simulink model "sampleModel347"  (R2021b)
settings: Solver=VariableStepAuto  StartTime=0.0  StopTime=10.0  RelTol=1e-3
undefined symbols (not defined in the file or in its folder): DiscIntNeverNeededParam, Newton, Raphson
libraries: simulink x9, slpidlib x1
settings Model: Creator=user  LastModifiedBy=user

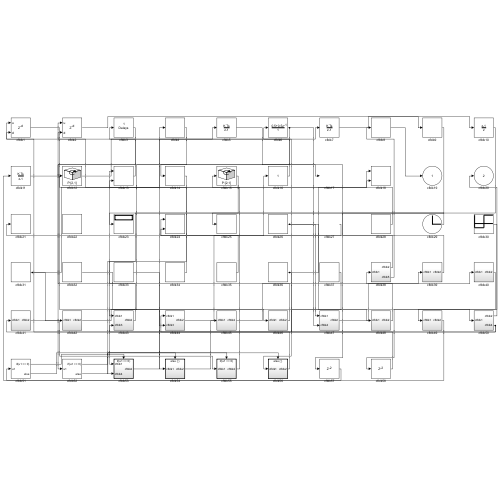
[thumbnail: Simulink's stored preview of the top-level diagram]
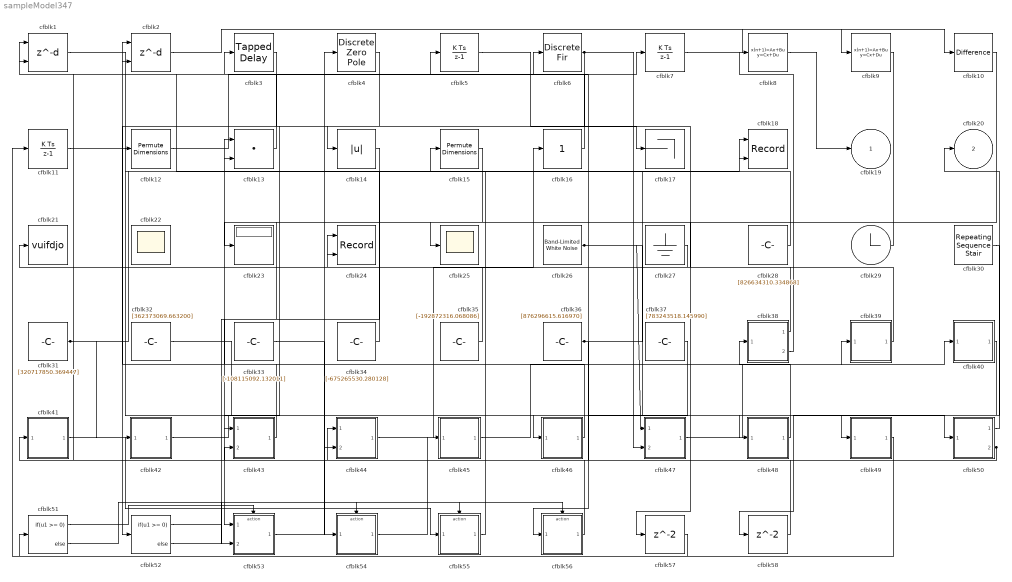
== system sampleModel347 ==
  cfblk1 : Delay  DelayLengthSource=Input port  SampleTime=1
      settings: InputPortMap=u0,p1
  cfblk10 : simulink/Discrete/Difference  ICPrevInput=0.0  OutMin=[]  OutMax=[]  OutDataTypeStr=Inherit: Inherit via back propagation  OutDataType=fixdt(1, 16)  OutScaling=2^-10  DoSatur=off
  cfblk11 : DiscreteIntegrator  ICPrevOutput=DiscIntNeverNeededParam  ICPrevScaledInput=DiscIntNeverNeededParam
  cfblk12 : PermuteDimensions
  cfblk13 : DotProduct  InputSameDT=on  OutDataTypeStr=Inherit: Inherit via internal rule
  cfblk14 : Abs
  cfblk15 : PermuteDimensions
  cfblk16 : simulink/Math Operations/Slider Gain  gain=1  low=0  high=2
  cfblk17 : Terminator
  cfblk18 : Record  FileSettingsInternal="{\"entries\":[{\"content\":{\"excelSettings\":{\"content\":{},\"type\":\"Streamout.ExcelSettings\"}},\"type\":\"Streamout.FileSettingStorage\",\"uuid\":\"55d644a5-12b3-4429-a882-e1257f208ec1\"}],\"packageUris\":[\"http://schema.mathworks.com/mf0/streamout_blocks/R2020a\"],\"version\":\"1.0\"}"  Layout=[1 1]  SignalsInternal="{\"entries\":[{\"content\":{\"signals\":[{\"content\":{\"blockPath\":[\"sampleModel347/cfblk18\"],\"channel\":[],\"dimensions\":[1],\"domain\":\"sampleModel347/cfblk18\",\"lineColor\":\"#a2142f\",\"plots\":[1],\"port\":1,\"sid\":[\"\"],\"signalID\":14541,\"signalName\":\"cfblk36\"},\"type\":\"RecordBlkView.Signal\",\"uuid\":\"b67f685b-2653-4f6a-806c-a94c2618ce46\"},{\"content\":{\"blockPath\":[\"sampleModel347/cfblk18\"],\"channel\":[],\"dimensions\":[1],\"domain\":\"sampleModel347/cfblk18\",\"lineColor\":\"#139fff\",\"plots\":[1],\"port\":2,\"sid\":[\"\"],\"signalID\":14545,\"signalName\":\"cfblk11\"},\"type\":\"RecordBlkView.Signal\",\"uuid\":\"4f3fc5b9-18d0-4829-bc90-462738cc687d\"}]},\"type\":\"RecordBlkView.InputSignals\",\"uuid\":\"f6bcba47-d682-4b72-9895-2afc48cdd87f\"}],\"packageUris\":[\"http://schema.mathworks.com/mf0/streamout_blocks/R2020a\"],\"version\":\"1.0\"}"  VisualizationBindings="{\"xyplotplugin\":{\"info\":[{\"series\":[{\"bindingParametersList\":[{\"parameter\":\"X-Axis\",\"signalID\":14541,\"signalName\":\"cfblk36\"},{\"parameter\":\"Y-Axis\",\"signalID\":14545,\"signalName\":\"cfblk11\"}],\"seriesID\":40911}],\"subplotID\":1}]}}"  CompatibilityTag=XY
  cfblk2 : Delay  DelayLengthSource=Input port  SampleTime=1
      settings: InputPortMap=u0,p1
  cfblk21 : ToWorkspace  VariableName=vuifdjo  SaveFormat=Timeseries  SampleTime=-1
  cfblk22 : Scope
      settings: Floating=on
  cfblk23 : Display
  cfblk24 : Record  FileSettingsInternal="{\"entries\":[{\"content\":{\"excelSettings\":{\"content\":{},\"type\":\"Streamout.ExcelSettings\"}},\"type\":\"Streamout.FileSettingStorage\",\"uuid\":\"c7d4169a-b585-49ac-aca8-b838ce6defab\"}],\"packageUris\":[\"http://schema.mathworks.com/mf0/streamout_blocks/R2020a\"],\"version\":\"1.0\"}"  Layout=[1 1]  SignalsInternal="{\"entries\":[{\"content\":{\"signals\":[{\"content\":{\"blockPath\":[\"sampleModel347/cfblk24\"],\"channel\":[],\"dimensions\":[1],\"domain\":\"sampleModel347/cfblk24\",\"lineColor\":\"#a2142f\",\"plots\":[1],\"port\":1,\"sid\":[\"\"],\"signalID\":14549,\"signalName\":\"cfblk35\"},\"type\":\"RecordBlkView.Signal\",\"uuid\":\"209a5a0c-6ba4-41ae-874b-22178ed96705\"},{\"content\":{\"blockPath\":[\"sampleModel347/cfblk24\"],\"channel\":[],\"dimensions\":[1],\"domain\":\"sampleModel347/cfblk24\",\"lineColor\":\"#139fff\",\"plots\":[1],\"port\":2,\"sid\":[\"\"],\"signalID\":14553,\"signalName\":\"cfblk27\"},\"type\":\"RecordBlkView.Signal\",\"uuid\":\"494a0b99-c67e-416d-8697-a0053402a19d\"}]},\"type\":\"RecordBlkView.InputSignals\",\"uuid\":\"05a8ac8a-22e6-46ac-8d63-08b6bf11da06\"}],\"packageUris\":[\"http://schema.mathworks.com/mf0/streamout_blocks/R2020a\"],\"version\":\"1.0\"}"  VisualizationBindings="{\"xyplotplugin\":{\"info\":[{\"series\":[{\"bindingParametersList\":[{\"parameter\":\"X-Axis\",\"signalID\":14549,\"signalName\":\"cfblk35\"},{\"parameter\":\"Y-Axis\",\"signalID\":14553,\"signalName\":\"cfblk27\"}],\"seriesID\":25638}],\"subplotID\":1}]}}"  CompatibilityTag=XY
  cfblk25 : Scope
  cfblk26 : simulink/Sources/Band-Limited White Noise  Cov=[3794398979.519006]  Ts=0.1  seed=[782136946.000000]
  cfblk27 : Ground
  cfblk28 : Constant  Value=[826634310.334868]  SampleTime=1
  cfblk29 : Clock
  cfblk3 : simulink/Discrete/Tapped Delay  vinit=0.0  samptime=-1  NumDelays=1  DelayOrder=Oldest  includeCurrent=off
  cfblk30 : simulink/Sources/Repeating Sequence Stair  OutValues=[-457308169.608421, 909466912.372640]  tsamp=-1  OutMin=[]  OutMax=[]  OutDataTypeStr=double  OutputDataTypeScalingMode=double  OutDataType=fixdt(0,8)  ConRadixGroup=Best Precision: Vector-wise  OutScaling=2^-12
  cfblk31 : Constant  Value=[320717850.369447]  SampleTime=1
  cfblk32 : Constant  Value=[362373069.663200]  SampleTime=1
  cfblk33 : Constant  Value=[-108115092.132011]  SampleTime=1
  cfblk34 : Constant  Value=[-675265530.280128]  SampleTime=1
  cfblk35 : Constant  Value=[-192872316.068086]  SampleTime=1
  cfblk36 : Constant  Value=[876296615.616970]  SampleTime=1
  cfblk37 : Constant  Value=[783243518.145990]  SampleTime=1
  cfblk38 : Subsystem
  cfblk39 : Subsystem
  cfblk4 : DiscreteZeroPole  Poles=[0 0.5]  Gain=1
  cfblk40 : Subsystem
  cfblk41 : Subsystem
  cfblk42 : Subsystem
  cfblk43 : Subsystem
  cfblk44 : Subsystem
  cfblk45 : Subsystem
  cfblk46 : Subsystem
  cfblk47 : Subsystem
  cfblk48 : Subsystem
  cfblk49 : Subsystem
  cfblk5 : DiscreteIntegrator  ICPrevOutput=DiscIntNeverNeededParam  ICPrevScaledInput=DiscIntNeverNeededParam
  cfblk50 : Subsystem
  cfblk51 : If  IfExpression=u1 >= 0  SampleTime=1
  cfblk52 : If  IfExpression=u1 >= 0  SampleTime=1
  cfblk53 : Subsystem  TreatAsAtomicUnit=on
  cfblk54 : Subsystem  TreatAsAtomicUnit=on
  cfblk55 : Subsystem  TreatAsAtomicUnit=on
  cfblk56 : Subsystem  TreatAsAtomicUnit=on
  cfblk57 : Delay  SampleTime=1
  cfblk58 : Delay  SampleTime=1
  cfblk6 : DiscreteFir  SampleTime=1
  cfblk7 : DiscreteIntegrator  ICPrevOutput=DiscIntNeverNeededParam  ICPrevScaledInput=DiscIntNeverNeededParam
  cfblk8 : DiscreteStateSpace
  cfblk9 : DiscreteStateSpace
  cfblk19 : Outport
  cfblk20 : Outport  Port=2
  wires:
  cfblk32/1 -> cfblk46/1(cfblk1)
  cfblk15/1 -> cfblk25/1
  cfblk37/1 -> cfblk44/1(cfblk1)
  cfblk35/1 -> cfblk24/1
  cfblk27/1 -> cfblk24/2
  cfblk38/1(cfblk2) -> cfblk14/1
  cfblk13/1 -> cfblk1/1
  cfblk1/1 -> cfblk44/2(cfblk3)
  cfblk16/1 -> cfblk3/1
  cfblk55/1(cfblk2) -> cfblk15/1
  cfblk36/1 -> cfblk18/1, cfblk56/1(cfblk1)
  cfblk26/1 -> cfblk47/1(cfblk1), cfblk50/1(cfblk1)
  cfblk33/1 -> cfblk54/1(cfblk1)
  cfblk12/1 -> cfblk5/1
  cfblk7/1 -> cfblk10/1
  cfblk4/1 -> cfblk52/1
  cfblk38/2(cfblk5) -> cfblk21/1
  cfblk5/1 -> cfblk17/1
  cfblk49/1(cfblk2) -> cfblk11/1
  cfblk46/1(cfblk2) -> cfblk13/1
  cfblk30/1 -> cfblk49/1(cfblk1)
  cfblk41/1(cfblk2) -> cfblk55/1(cfblk1)
  cfblk6/1 -> cfblk47/2(cfblk4), cfblk43/1(cfblk1)
  cfblk31/1 -> cfblk4/1, cfblk42/1(cfblk1)
  cfblk53/1(cfblk2) -> cfblk7/1
  cfblk39/1(cfblk2) -> cfblk8/1
  cfblk56/1(cfblk2) -> cfblk1/2
  cfblk44/1(cfblk2) -> cfblk16/1
  cfblk8/1 -> cfblk19/1
  cfblk28/1 -> cfblk13/2
  cfblk54/1(cfblk2) -> cfblk45/1(cfblk1)
  cfblk29/1 -> cfblk23/1
  cfblk11/1 -> cfblk18/2
  cfblk47/1(cfblk2) -> cfblk40/1(cfblk1)
  cfblk2/1 -> cfblk9/1
  cfblk43/1(cfblk2) -> cfblk2/1
  cfblk3/1 -> cfblk12/1
  cfblk9/1 -> cfblk53/1(cfblk1)
  cfblk14/1 -> cfblk53/2(cfblk4)
  cfblk42/1(cfblk2) -> cfblk48/1(cfblk1)
  cfblk34/1 -> cfblk2/2
  cfblk48/1(cfblk2) -> cfblk38/1(cfblk1)
  cfblk45/1(cfblk2) -> cfblk39/1(cfblk1)
  cfblk50/1(cfblk2) -> cfblk20/1
  cfblk50/2(cfblk4) -> cfblk41/1(cfblk1), cfblk43/2(cfblk3)
  cfblk51/1 -> cfblk53/Action
  cfblk51/2 -> cfblk54/Action
  cfblk52/1 -> cfblk55/Action
  cfblk52/2 -> cfblk56/Action
  cfblk10/1 -> cfblk57/1
  cfblk57/1 -> cfblk51/1
  cfblk40/1(cfblk2) -> cfblk58/1
  cfblk58/1 -> cfblk6/1

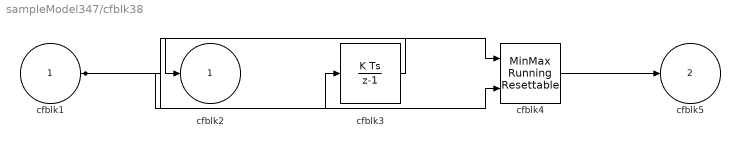
== system sampleModel347/cfblk38 ==
  cfblk1 : Inport
  cfblk3 : DiscreteIntegrator  ICPrevOutput=DiscIntNeverNeededParam  ICPrevScaledInput=DiscIntNeverNeededParam
  cfblk4 : simulink/Math Operations/MinMax Running Resettable  Function=min  vinit=0.0
  cfblk2 : Outport
  cfblk5 : Outport  Port=2
  wires:
  cfblk3/1 -> cfblk2/1
  cfblk1/1 -> cfblk3/1, cfblk4/1, cfblk4/2
  cfblk4/1 -> cfblk5/1

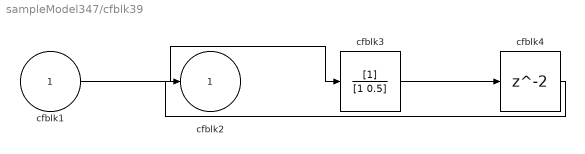
== system sampleModel347/cfblk39 ==
  cfblk1 : Inport
  cfblk3 : DiscreteFilter  SampleTime=1
  cfblk4 : Delay  SampleTime=1
  cfblk2 : Outport
  wires:
  cfblk3/1 -> cfblk4/1
  cfblk1/1 -> cfblk3/1
  cfblk4/1 -> cfblk2/1

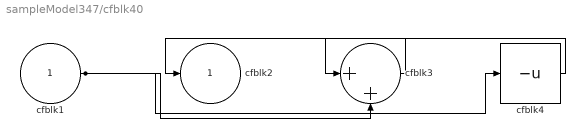
== system sampleModel347/cfblk40 ==
  cfblk1 : Inport
  cfblk3 : Sum  Inputs=|++
  cfblk4 : UnaryMinus
  cfblk2 : Outport
  wires:
  cfblk3/1 -> cfblk2/1
  cfblk1/1 -> cfblk4/1, cfblk3/2
  cfblk4/1 -> cfblk3/1

== system sampleModel347/cfblk41 ==
  cfblk1 : Inport
  cfblk3 : UnaryMinus
  cfblk2 : Outport
  wires:
  cfblk1/1 -> cfblk3/1
  cfblk3/1 -> cfblk2/1

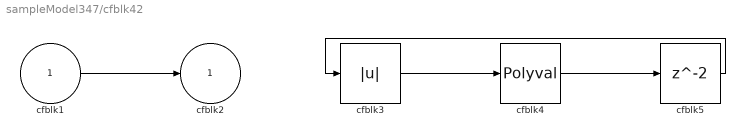
== system sampleModel347/cfblk42 ==
  cfblk1 : Inport
  cfblk3 : Abs
  cfblk4 : Polyval  Coefs=[ +2.081618890e-019, -1.441693666e-014, +4.719686976e-010, -8.536869453e-006, +1.621573104e-001, -8.087801117e+001 ]
  cfblk5 : Delay  SampleTime=1
  cfblk2 : Outport
  wires:
  cfblk1/1 -> cfblk2/1
  cfblk3/1 -> cfblk4/1
  cfblk4/1 -> cfblk5/1
  cfblk5/1 -> cfblk3/1

== system sampleModel347/cfblk43 ==
  cfblk1 : Inport
  cfblk3 : Inport  Port=2
  cfblk2 : Outport
  wires:
  cfblk3/1 -> cfblk2/1

== system sampleModel347/cfblk44 ==
  cfblk1 : Inport
  cfblk3 : Inport  Port=2
  cfblk2 : Outport
  wires:
  cfblk3/1 -> cfblk2/1

== system sampleModel347/cfblk45 ==
  cfblk1 : Inport
  cfblk3 : Sqrt  Operator=rSqrt  AlgorithmType=Newton-Raphson  SaturateOnIntegerOverflow=on
  cfblk2 : Outport
  wires:
  cfblk1/1 -> cfblk3/1
  cfblk3/1 -> cfblk2/1

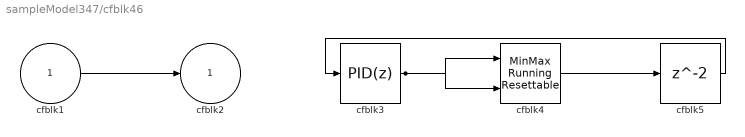
== system sampleModel347/cfblk46 ==
  cfblk1 : Inport
  cfblk3 : slpidlib/PID Controller  Controller=PID  Form=Parallel  TimeDomain=Discrete-time  UseExternalTs=off  SampleTime=1  IntegratorMethod=Forward Euler  FilterMethod=Forward Euler  ControllerParametersSource=internal  P=1  I=1  D=0  UseFilter=on  N=100  TunerSelectOption=Transfer Function Based (PID Tuner App)  InitialConditionSource=internal  InitialConditionForIntegrator=0  InitialConditionForFilter=0  DifferentiatorICPrevScaledInput=0  ExternalReset=none  TrackingMode=off  Kt=1  LimitOutput=off  SatLimitsSource=internal  UpperSaturationLimit=inf  LowerSaturationLimit=-inf  LinearizeAsGain=off  AntiWindupMode=none  Kb=1  POutMin=[]  POutMax=[]  IOutMin=[]  IOutMax=[]  DOutMin=[]  DOutMax=[]  NOutMin=[]  NOutMax=[]  SumOutMin=[]  SumOutMax=[]  SaturationOutMin=[]  SaturationOutMax=[]  PParamMin=[]  PParamMax=[]  IParamMin=[]  IParamMax=[]  DParamMin=[]  DParamMax=[]  NParamMin=[]  NParamMax=[]  KbParamMin=[]  KbParamMax=[]  KtParamMin=[]  KtParamMax=[]  KbOutMin=[]  KbOutMax=[]  KtOutMin=[]  KtOutMax=[]  IntegratorOutMin=[]  IntegratorOutMax=[]  FilterOutMin=[]  FilterOutMax=[]  SumI1OutMin=[]  SumI1OutMax=[]  SumI2OutMin=[]  SumI2OutMax=[]  SumI3OutMin=[]  SumI3OutMax=[]  SumI4OutMin=[]  SumI4OutMax=[]  SumDOutMin=[]  SumDOutMax=[]  DifferentiatorOutMin=[]  DifferentiatorOutMax=[]  FilterDiffOutCoefMin=[]  FilterDiffOutCoefMax=[]  ReciprocalOutMin=[]  ReciprocalOutMax=[]  SumDenOutMin=[]  SumDenOutMax=[]  SumNumOutMin=[]  SumNumOutMax=[]  DivideOutMin=[]  DivideOutMax=[]  UdiffTsProdOutMin=[]  UdiffTsProdOutMax=[]  NTsProdOutMin=[]  NTsProdOutMax=[]  UintegralTsProdOutMin=[]  UintegralTsProdOutMax=[]  UngainTsProdOutMin=[]  UngainTsProdOutMax=[]  IntegratorContinuousStateAttributes=''  IntegratorStateMustResolveToSignalObject=off  IntegratorRTWStateStorageClass=Auto  FilterContinuousStateAttributes=''  FilterStateMustResolveToSignalObject=off  FilterRTWStateStorageClass=Auto  ParallelPVariant=InternalParameters  IdealPVariant=Disabled  IVariant=InternalParameters  DVariant=InternalParameters  IntegratorVariant=Discrete  SatVariant=Disabled  AWVariant=Passthrough  PCopyVariant=Disabled  TRVariant=Disabled  FdbkBlocksVariant=Forward  IdealPFdbkVariant=Disabled  SatFdbkVariant=Disabled  DerivativeFilterVariant=ForwardEulerFilter  NVariant=InternalParameters  NCopyVariant=Disabled  FilterICVariant=InternalICsFilter  IntegratorICVariant=InternalICs  ExternalResetVariant=Disabled  TRSumVariant=Passthrough  SumFdbkVariant=Disabled  SumVariant=Sum_PID  TsampFilterVariant=InternalTs  TsampNgainVariant=Passthrough  TsampIntegralVariant=Passthrough  ExternalSaturationOutDataTypeStr=Inherit: Same as second input
  cfblk4 : simulink/Math Operations/MinMax Running Resettable  Function=min  vinit=0.0
  cfblk5 : Delay  SampleTime=1
  cfblk2 : Outport
  wires:
  cfblk1/1 -> cfblk2/1
  cfblk3/1 -> cfblk4/1, cfblk4/2
  cfblk4/1 -> cfblk5/1
  cfblk5/1 -> cfblk3/1

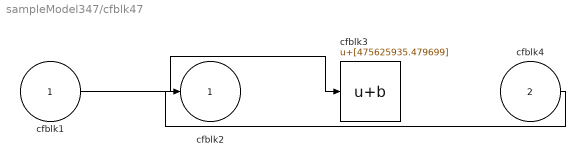
== system sampleModel347/cfblk47 ==
  cfblk1 : Inport
  cfblk4 : Inport  Port=2
  cfblk3 : Bias  Bias=[475625935.479699]
  cfblk2 : Outport
  wires:
  cfblk1/1 -> cfblk3/1
  cfblk4/1 -> cfblk2/1

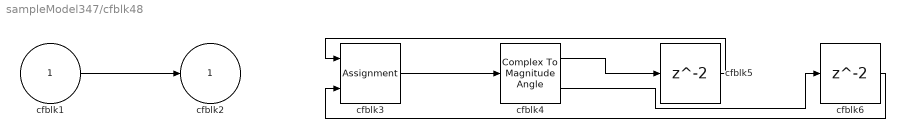
== system sampleModel347/cfblk48 ==
  cfblk1 : Inport
  cfblk3 : Assignment  DiagnosticForDimensions=Warning  IndexOptions=Index vector (dialog)  Indices=1  OutputSizes=1
  cfblk4 : ComplexToMagnitudeAngle
  cfblk5 : Delay  SampleTime=1
  cfblk6 : Delay  SampleTime=1
  cfblk2 : Outport
  wires:
  cfblk1/1 -> cfblk2/1
  cfblk3/1 -> cfblk4/1
  cfblk4/1 -> cfblk5/1
  cfblk5/1 -> cfblk3/1
  cfblk4/2 -> cfblk6/1
  cfblk6/1 -> cfblk3/2

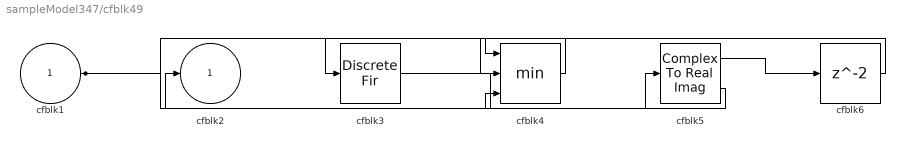
== system sampleModel347/cfblk49 ==
  cfblk1 : Inport
  cfblk3 : DiscreteFir  SampleTime=1
  cfblk4 : MinMax  Inputs=3
  cfblk5 : ComplexToRealImag
  cfblk6 : Delay  SampleTime=1
  cfblk2 : Outport
  wires:
  cfblk5/2 -> cfblk2/1
  cfblk3/1 -> cfblk5/1
  cfblk4/1 -> cfblk3/1
  cfblk1/1 -> cfblk4/2, cfblk4/3
  cfblk5/1 -> cfblk6/1
  cfblk6/1 -> cfblk4/1

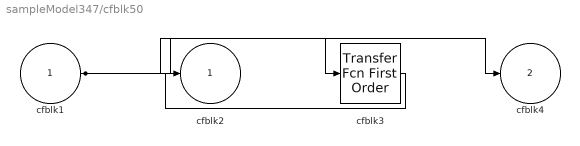
== system sampleModel347/cfblk50 ==
  cfblk1 : Inport
  cfblk3 : simulink/Discrete/Transfer Fcn First Order  PoleZ=0.95  ICPrevOutput=0.0  DoSatur=off
  cfblk2 : Outport
  cfblk4 : Outport  Port=2
  wires:
  cfblk1/1 -> cfblk4/1, cfblk3/1
  cfblk3/1 -> cfblk2/1

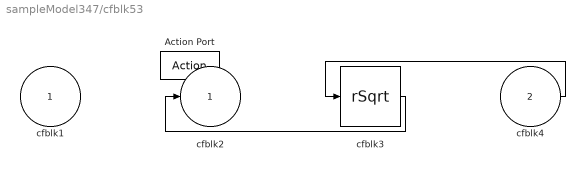
== system sampleModel347/cfblk53 ==
  cfblk1 : Inport
  cfblk4 : Inport  Port=2
  Action Port : ActionPort  ActionPortLabel=if(u1 >= 0)
  cfblk3 : Sqrt  Operator=rSqrt  AlgorithmType=Newton-Raphson  SaturateOnIntegerOverflow=on
  cfblk2 : Outport
  wires:
  cfblk4/1 -> cfblk3/1
  cfblk3/1 -> cfblk2/1

== system sampleModel347/cfblk54 ==
  cfblk1 : Inport
  Action Port : ActionPort  ActionPortLabel=else
  cfblk3 : simulink/Discrete/Tapped Delay  vinit=0.0  samptime=-1  NumDelays=1  DelayOrder=Oldest  includeCurrent=off
  cfblk2 : Outport
  wires:
  cfblk3/1 -> cfblk2/1
  cfblk1/1 -> cfblk3/1

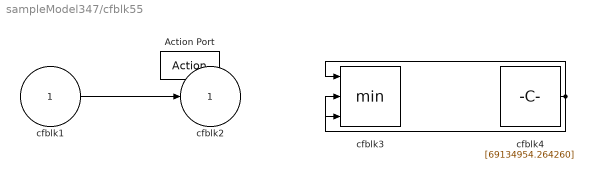
== system sampleModel347/cfblk55 ==
  cfblk1 : Inport
  Action Port : ActionPort  ActionPortLabel=if(u1 >= 0)
  cfblk3 : MinMax  Inputs=3
  cfblk4 : Constant  Value=[69134954.264260]  SampleTime=1
  cfblk2 : Outport
  wires:
  cfblk1/1 -> cfblk2/1
  cfblk4/1 -> cfblk3/1, cfblk3/2, cfblk3/3

== system sampleModel347/cfblk56 ==
  cfblk1 : Inport
  Action Port : ActionPort  ActionPortLabel=else
  cfblk3 : UnitDelay  SampleTime=-1  HasFrameUpgradeWarning=on
  cfblk2 : Outport
  wires:
  cfblk1/1 -> cfblk2/1, cfblk3/1
